simulink model "simulation_Hippocampus_compare_paper"  (R2023a)
settings: Solver=ode3  StartTime=0  StopTime=120  FixedStep=0.001  MaxStep=0.001  MinStep=0.00001  RelTol=1e-5  AbsTol=1e-5  EnableMultiTasking=on
values from neighbouring files (symbols this model uses):
  k_pos_ndi = 8    [parameters.m]
  k_vel_ndi = 8    [parameters.m]
  Kf = 6    [parameters.m]
  Kp = 0.01    [parameters.m]
  Kp_p = 30    [parameters.m]
  Kp_pitch = 8    [parameters.m]
  Kp_q = 10    [parameters.m]
  Kp_r = 10    [parameters.m]
  Kp_roll = 10    [parameters.m]
  Kp_u = 8    [parameters.m]
  Kp_yaw = 8    [parameters.m]
  Kq = 5    [parameters.m]
  Kr = 8    [parameters.m]
  Ktau1 = 0.1    [parameters.m]
  Ktau2 = 5    [parameters.m]
  Ktau3 = 5    [parameters.m]
  Ku = 8    [parameters.m]
  p11 = 0.4    [parameters.m]
  p12 = 0.2    [parameters.m]
  p21 = 0.2    [parameters.m]
  p22 = 0.05    [parameters.m]
  p31 = 0.3    [parameters.m]
  p32 = 0.05    [parameters.m]
  p41 = 0.5    [parameters.m]
  p42 = 0.1    [parameters.m]
  p51 = 0.5    [parameters.m]
  p52 = 0.1    [parameters.m]
  p61 = 0.5    [parameters.m]
  p62 = 0.1    [parameters.m]
  Q1 = -8    [simulation_para.m]
  Q2 = -10    [simulation_para.m]
  Q3 = -[0.01,5,8]    [simulation_para.m]
  Q4 = -[0.001,0.1,0.1]    [simulation_para.m]
  r1 = 4    [parameters.m]
  r2 = 6    [parameters.m]
libraries: simulink x8
(part 2 of 7)

== system simulation_Hippocampus_compare_paper/PDPD1/HippCampus1 ==
  input : Inport
  disturbance : Inport  Port=2
  Controls: Angular Velocities : Scope
  Controls: Rotors1 : Scope
  Controls: Torques : Scope
  Display : Display
  Display1 : Display
  HippoCampus : MATLAB Function  TreatAsAtomicUnit=on
  Integrator : Integrator  InitialCondition=[0; 0; 0; 0;0;0;zeros(6,1)]
  Subsystem : Subsystem
  Subsystem1 : Subsystem
  Subsystem4 : Subsystem
  Sum : Sum  Inputs=|++
  To Workspace8 : ToWorkspace  VariableName=u_PDPD  SaveFormat=Timeseries  SampleTime=-1
  state : Outport
  wires:
  HippoCampus/1(dx) -> Sum/1  "dx"
  Sum/1 -> Integrator/1
  ? -> Controls: Angular Velocities/1
  disturbance/1 -> Sum/2
  Integrator/1 -> Subsystem/1(In1)
  Subsystem/1(state) -> state/1, HippoCampus/1(x)
  Subsystem4/1(Out1) -> Display1/1
  Subsystem1/1(Out1) -> Display/1
  input/1 -> Subsystem4/1(u), To Workspace8/1, Subsystem1/1(u), HippoCampus/2(in), Controls: Torques/1, Controls: Rotors1/1

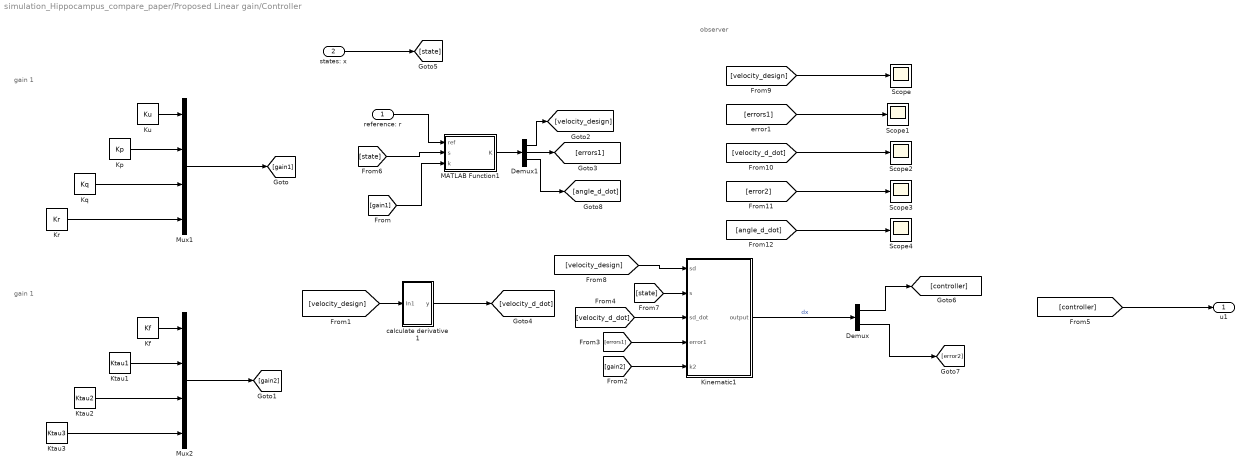
== system simulation_Hippocampus_compare_paper/Proposed Linear gain/Controller ==
  note: observer
  note: gain 1
  note: gain 1
  reference: r : Inport
  states: x : Inport  Port=2
  Demux : Demux  Outputs=[4 4]
  Demux1 : Demux  Outputs=[4 4 2]
  Kf : Constant  Value=Kf
  Kinematic1 : MATLAB Function  TreatAsAtomicUnit=on
  Kp : Constant  Value=Kp
  Kq : Constant  Value=Kq
  Kr : Constant  Value=Kr
  Ktau1 : Constant  Value=Ktau1
  Ktau2 : Constant  Value=Ktau2
  Ktau3 : Constant  Value=Ktau3
  Ku : Constant  Value=Ku
  MATLAB Function1 : MATLAB Function  TreatAsAtomicUnit=on
  Mux1 : Mux
  Mux2 : Mux
  Scope{,1..4} (5 alike) : Scope
  calculate derivative 1 : Subsystem
  u1 : Outport
  wires:
  Kinematic1/1(output) -> Demux/1  "dx"
  [state] -> Kinematic1/2(s)
  reference: r/1 -> MATLAB Function1/1(ref)
  states: x/1 -> [state]
  Ku/1 -> Mux1/1
  Kp/1 -> Mux1/2
  Kq/1 -> Mux1/3
  Kr/1 -> Mux1/4
  Mux1/1 -> [gain1]
  [gain1] -> MATLAB Function1/3(k)
  Ktau3/1 -> Mux2/4
  Ktau1/1 -> Mux2/2
  Ktau2/1 -> Mux2/3
  Mux2/1 -> [gain2]
  Kf/1 -> Mux2/1
  Demux1/1 -> [velocity_design]
  MATLAB Function1/1(K) -> Demux1/1
  Demux1/2 -> [errors1]
  [velocity_design] -> calculate derivative 1/1(In1)
  [gain2] -> Kinematic1/5(k2)
  [errors1] -> Kinematic1/4(error1)
  [state] -> MATLAB Function1/2(s)
  [velocity_design] -> Kinematic1/1(sd)
  Demux/1 -> [controller]
  Demux/2 -> [error2]
  [controller] -> u1/1
  [velocity_design] -> Scope/1
  [errors1] -> Scope1/1
  [velocity_d_dot] -> Scope2/1
  [error2] -> Scope3/1
  calculate derivative 1/1(y) -> [velocity_d_dot]
  Demux1/3 -> [angle_d_dot]
  [angle_d_dot] -> Scope4/1
  [velocity_d_dot] -> Kinematic1/3(sd_dot)

== system simulation_Hippocampus_compare_paper/Proposed Linear gain/Disturbance: All derivatives1 ==
  a : Inport
  a1 : Inport  Port=2
  Input : Inport  Port=3
  Gain1 : Gain  Gain=0  Multiplication=Matrix(K*u)
  Gain2 : Gain  Multiplication=Matrix(K*u)
  Gain3 : Gain  Gain=0  Multiplication=Matrix(K*u)
  MATLAB Function : MATLAB Function  TreatAsAtomicUnit=on
  Sum2 : Sum  Inputs=|+++
  disturbance2 : Subsystem
  disturbance3 : Subsystem
  old disturbance : Subsystem
  disturbance : Outport
  wires:
  Sum2/1 -> MATLAB Function/1(u)
  Gain1/1 -> Sum2/1
  disturbance2/1(Out1) -> Gain2/1
  a/1 -> disturbance3/1(a)
  a1/1 -> disturbance3/2(a1)
  disturbance3/1(d) -> Gain1/1
  Gain2/1 -> Sum2/2
  old disturbance/1(Out1) -> Gain3/1
  Gain3/1 -> Sum2/3
  MATLAB Function/1(y) -> disturbance/1
  Input/1 -> MATLAB Function/2(d)

== system simulation_Hippocampus_compare_paper/Proposed Linear gain/Disturbance: All derivatives2 ==
  a : Inport
  a1 : Inport  Port=2
  Input : Inport  Port=3
  Input1 : Inport  Port=4
  Gain1 : Gain  Gain=0  Multiplication=Matrix(K*u)
  Gain2 : Gain  Multiplication=Matrix(K*u)
  Gain3 : Gain  Gain=0  Multiplication=Matrix(K*u)
  Gain4 : Gain  Gain=0  Multiplication=Matrix(K*u)
  MATLAB Function : MATLAB Function  TreatAsAtomicUnit=on
  MATLAB Function1 : MATLAB Function  TreatAsAtomicUnit=on
  Scope : Scope
  Sum2 : Sum  Inputs=|++++
  disturbance2 : Subsystem
  disturbance3 : Subsystem
  old disturbance : Subsystem
  disturbance : Outport
  wires:
  Sum2/1 -> MATLAB Function/1(u)
  Gain1/1 -> Sum2/1
  disturbance2/1(Out1) -> Gain2/1
  a/1 -> disturbance3/1(a)
  a1/1 -> disturbance3/2(a1)
  disturbance3/1(d) -> Gain1/1
  Gain2/1 -> Sum2/2
  old disturbance/1(Out1) -> Gain3/1
  Gain3/1 -> Sum2/3
  MATLAB Function/1(y) -> disturbance/1
  Input/1 -> MATLAB Function/2(d)
  Input1/1 -> MATLAB Function1/1(u)
  MATLAB Function1/1(d) -> Scope/1, Gain4/1
  Gain4/1 -> Sum2/4

== system simulation_Hippocampus_compare_paper/Proposed Linear gain/HippCampus ==
  input : Inport
  disturbance : Inport  Port=2
  Controls: Rotors1 : Scope
  Controls: Torques : Scope
  Display : Display
  Display1 : Display
  HippoCampus : MATLAB Function  TreatAsAtomicUnit=on
  Integrator : Integrator  InitialCondition=[0; 0; 0; 0;0;0;zeros(6,1)]
  Scope : Scope
  Subsystem : Subsystem
  Subsystem1 : Subsystem
  Subsystem4 : Subsystem
  Sum : Sum  Inputs=|++
  To Workspace7 : ToWorkspace  VariableName=LYAL_u  SaveFormat=Timeseries  SampleTime=-1
  sat1 : MATLAB Function  TreatAsAtomicUnit=on
  state : Outport
  wires:
  HippoCampus/1(dx) -> Sum/1  "dx"
  Sum/1 -> Integrator/1
  disturbance/1 -> Sum/2
  Integrator/1 -> Subsystem/1(In1)
  Subsystem/1(state) -> state/1, HippoCampus/1(x)
  Subsystem4/1(Out1) -> Display1/1
  Subsystem1/1(Out1) -> Display/1
  sat1/1(u_sat) -> Controls: Rotors1/1, Controls: Torques/1, Scope/1, HippoCampus/2(in), Subsystem1/1(u), Subsystem4/1(u), To Workspace7/1
  input/1 -> sat1/1(u)

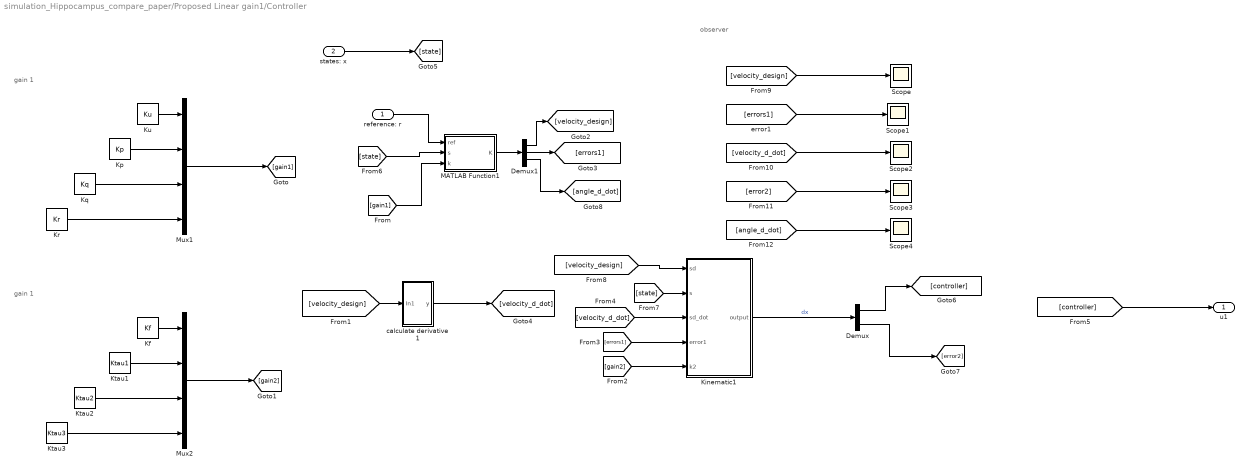
== system simulation_Hippocampus_compare_paper/Proposed Linear gain1/Controller ==
  note: observer
  note: gain 1
  note: gain 1
  reference: r : Inport
  states: x : Inport  Port=2
  Demux : Demux  Outputs=[4 4]
  Demux1 : Demux  Outputs=[4 4 2]
  Kf : Constant  Value=Kf
  Kinematic1 : MATLAB Function  TreatAsAtomicUnit=on
  Kp : Constant  Value=Kp
  Kq : Constant  Value=Kq
  Kr : Constant  Value=Kr
  Ktau1 : Constant  Value=Ktau1
  Ktau2 : Constant  Value=Ktau2
  Ktau3 : Constant  Value=Ktau3
  Ku : Constant  Value=Ku
  MATLAB Function1 : MATLAB Function  TreatAsAtomicUnit=on
  Mux1 : Mux
  Mux2 : Mux
  Scope{,1..4} (5 alike) : Scope
  calculate derivative 1 : Subsystem
  u1 : Outport
  wires:
  Kinematic1/1(output) -> Demux/1  "dx"
  [state] -> Kinematic1/2(s)
  reference: r/1 -> MATLAB Function1/1(ref)
  states: x/1 -> [state]
  Ku/1 -> Mux1/1
  Kp/1 -> Mux1/2
  Kq/1 -> Mux1/3
  Kr/1 -> Mux1/4
  Mux1/1 -> [gain1]
  [gain1] -> MATLAB Function1/3(k)
  Ktau3/1 -> Mux2/4
  Ktau1/1 -> Mux2/2
  Ktau2/1 -> Mux2/3
  Mux2/1 -> [gain2]
  Kf/1 -> Mux2/1
  Demux1/1 -> [velocity_design]
  MATLAB Function1/1(K) -> Demux1/1
  Demux1/2 -> [errors1]
  [velocity_design] -> calculate derivative 1/1(In1)
  [gain2] -> Kinematic1/5(k2)
  [errors1] -> Kinematic1/4(error1)
  [state] -> MATLAB Function1/2(s)
  [velocity_design] -> Kinematic1/1(sd)
  Demux/1 -> [controller]
  Demux/2 -> [error2]
  [controller] -> u1/1
  [velocity_design] -> Scope/1
  [errors1] -> Scope1/1
  [velocity_d_dot] -> Scope2/1
  [error2] -> Scope3/1
  calculate derivative 1/1(y) -> [velocity_d_dot]
  Demux1/3 -> [angle_d_dot]
  [angle_d_dot] -> Scope4/1
  [velocity_d_dot] -> Kinematic1/3(sd_dot)

== system simulation_Hippocampus_compare_paper/Proposed Linear gain1/Disturbance: All derivatives1 ==
  a : Inport
  a1 : Inport  Port=2
  Input : Inport  Port=3
  Gain1 : Gain  Gain=0  Multiplication=Matrix(K*u)
  Gain2 : Gain  Multiplication=Matrix(K*u)
  Gain3 : Gain  Gain=0  Multiplication=Matrix(K*u)
  MATLAB Function : MATLAB Function  TreatAsAtomicUnit=on
  Sum2 : Sum  Inputs=|+++
  disturbance2 : Subsystem
  disturbance3 : Subsystem
  old disturbance : Subsystem
  disturbance : Outport
  wires:
  Sum2/1 -> MATLAB Function/1(u)
  Gain1/1 -> Sum2/1
  disturbance2/1(Out1) -> Gain2/1
  a/1 -> disturbance3/1(a)
  a1/1 -> disturbance3/2(a1)
  disturbance3/1(d) -> Gain1/1
  Gain2/1 -> Sum2/2
  old disturbance/1(Out1) -> Gain3/1
  Gain3/1 -> Sum2/3
  MATLAB Function/1(y) -> disturbance/1
  Input/1 -> MATLAB Function/2(d)

== system simulation_Hippocampus_compare_paper/Proposed Linear gain1/HippCampus ==
  input : Inport
  disturbance : Inport  Port=2
  Controls: Rotors1 : Scope
  Controls: Torques : Scope
  Display : Display
  Display1 : Display
  HippoCampus : MATLAB Function  TreatAsAtomicUnit=on
  Integrator : Integrator  InitialCondition=[0; 0; 0; 0;0;0;zeros(6,1)]
  Scope : Scope
  Subsystem : Subsystem
  Subsystem1 : Subsystem
  Subsystem4 : Subsystem
  Sum : Sum  Inputs=|++
  To Workspace7 : ToWorkspace  VariableName=LYAL_u  SaveFormat=Timeseries  SampleTime=-1
  state : Outport
  wires:
  HippoCampus/1(dx) -> Sum/1  "dx"
  Sum/1 -> Integrator/1
  disturbance/1 -> Sum/2
  Integrator/1 -> Subsystem/1(In1)
  Subsystem/1(state) -> state/1, HippoCampus/1(x)
  Subsystem4/1(Out1) -> Display1/1
  Subsystem1/1(Out1) -> Display/1
  input/1 -> Controls: Rotors1/1, Controls: Torques/1, Scope/1, HippoCampus/2(in), Subsystem1/1(u), Subsystem4/1(u), To Workspace7/1

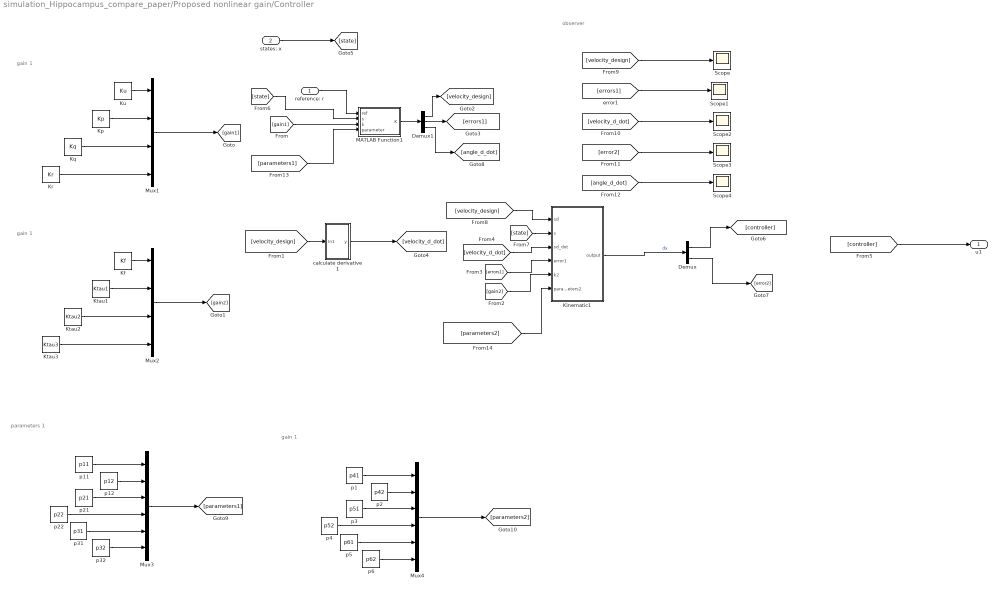
== system simulation_Hippocampus_compare_paper/Proposed nonlinear gain/Controller ==
  note: observer
  note: gain 1
  note: gain 1
  note: parameters 1
  note: gain 1
  reference: r : Inport
  states: x : Inport  Port=2
  Demux : Demux  Outputs=[4 4]
  Demux1 : Demux  Outputs=[4 4 2]
  Kf : Constant  Value=Kf
  Kinematic1 : MATLAB Function  TreatAsAtomicUnit=on
  Kp : Constant  Value=Kp
  Kq : Constant  Value=Kq
  Kr : Constant  Value=Kr
  Ktau1 : Constant  Value=Ktau1
  Ktau2 : Constant  Value=Ktau2
  Ktau3 : Constant  Value=Ktau3
  Ku : Constant  Value=Ku
  MATLAB Function1 : MATLAB Function  TreatAsAtomicUnit=on
  Mux1 : Mux
  Mux2 : Mux
  Mux3 : Mux  Inputs=6
  Mux4 : Mux  Inputs=6
  Scope{,1..4} (5 alike) : Scope
  calculate derivative 1 : Subsystem
  p1 : Constant  Value=p41
  p11 : Constant  Value=p11
  p12 : Constant  Value=p12
  p2 : Constant  Value=p42
  p21 : Constant  Value=p21
  p22 : Constant  Value=p22
  p3 : Constant  Value=p51
  p31 : Constant  Value=p31
  p32 : Constant  Value=p32
  p4 : Constant  Value=p52
  p5 : Constant  Value=p61
  p6 : Constant  Value=p62
  u1 : Outport
  wires:
  Kinematic1/1(output) -> Demux/1  "dx"
  [state] -> Kinematic1/2(s)
  reference: r/1 -> MATLAB Function1/1(ref)
  states: x/1 -> [state]
  Ku/1 -> Mux1/1
  Kp/1 -> Mux1/2
  Kq/1 -> Mux1/3
  Kr/1 -> Mux1/4
  Mux1/1 -> [gain1]
  [gain1] -> MATLAB Function1/3(k)
  Ktau3/1 -> Mux2/4
  Ktau1/1 -> Mux2/2
  Ktau2/1 -> Mux2/3
  Mux2/1 -> [gain2]
  Kf/1 -> Mux2/1
  Demux1/1 -> [velocity_design]
  MATLAB Function1/1(K) -> Demux1/1
  Demux1/2 -> [errors1]
  [velocity_design] -> calculate derivative 1/1(In1)
  [gain2] -> Kinematic1/5(k2)
  [errors1] -> Kinematic1/4(error1)
  [state] -> MATLAB Function1/2(s)
  [velocity_design] -> Kinematic1/1(sd)
  Demux/1 -> [controller]
  Demux/2 -> [error2]
  [controller] -> u1/1
  [velocity_design] -> Scope/1
  [errors1] -> Scope1/1
  [velocity_d_dot] -> Scope2/1
  [error2] -> Scope3/1
  calculate derivative 1/1(y) -> [velocity_d_dot]
  Demux1/3 -> [angle_d_dot]
  [angle_d_dot] -> Scope4/1
  [velocity_d_dot] -> Kinematic1/3(sd_dot)
  p22/1 -> Mux3/4
  p12/1 -> Mux3/2
  p21/1 -> Mux3/3
  Mux3/1 -> [parameters1]
  p11/1 -> Mux3/1
  p31/1 -> Mux3/5
  p32/1 -> Mux3/6
  [parameters1] -> MATLAB Function1/4(parameter)
  Mux4/1 -> [parameters2]
  p5/1 -> Mux4/5
  p6/1 -> Mux4/6
  p3/1 -> Mux4/3
  p2/1 -> Mux4/2
  p4/1 -> Mux4/4
  p1/1 -> Mux4/1
  [parameters2] -> Kinematic1/6(parameters2)

== system simulation_Hippocampus_compare_paper/Proposed nonlinear gain/Disturbance: All derivatives1 ==
  a : Inport
  a1 : Inport  Port=2
  Input : Inport  Port=3
  Input1 : Inport  Port=4
  Gain1 : Gain  Gain=0  Multiplication=Matrix(K*u)
  Gain2 : Gain  Multiplication=Matrix(K*u)
  Gain3 : Gain  Gain=0  Multiplication=Matrix(K*u)
  Gain4 : Gain  Gain=0  Multiplication=Matrix(K*u)
  MATLAB Function : MATLAB Function  TreatAsAtomicUnit=on
  MATLAB Function1 : MATLAB Function  TreatAsAtomicUnit=on
  Scope : Scope
  Sum2 : Sum  Inputs=|++++
  disturbance2 : Subsystem
  disturbance3 : Subsystem
  old disturbance : Subsystem
  disturbance : Outport
  wires:
  Sum2/1 -> MATLAB Function/1(u)
  Gain1/1 -> Sum2/1
  disturbance2/1(Out1) -> Gain2/1
  a/1 -> disturbance3/1(a)
  a1/1 -> disturbance3/2(a1)
  disturbance3/1(d) -> Gain1/1
  Gain2/1 -> Sum2/2
  old disturbance/1(Out1) -> Gain3/1
  Gain3/1 -> Sum2/3
  MATLAB Function/1(y) -> disturbance/1
  Input/1 -> MATLAB Function/2(d)
  Input1/1 -> MATLAB Function1/1(u)
  MATLAB Function1/1(d) -> Scope/1, Gain4/1
  Gain4/1 -> Sum2/4

== system simulation_Hippocampus_compare_paper/Proposed nonlinear gain/HippCampus ==
  input : Inport
  disturbance : Inport  Port=2
  Controls: Angular Velocities : Scope
  Controls: Rotors1 : Scope
  Controls: Torques : Scope
  Display : Display
  Display1 : Display
  HippoCampus : MATLAB Function  TreatAsAtomicUnit=on
  Integrator : Integrator  InitialCondition=[0; 0; 0; 0;0;0;zeros(6,1)]
  Scope : Scope
  Scope1 : Scope
  Subsystem : Subsystem
  Subsystem1 : Subsystem
  Subsystem4 : Subsystem
  Sum : Sum  Inputs=|++
  To Workspace7 : ToWorkspace  VariableName=u  SaveFormat=Timeseries  SampleTime=-1
  sat1 : MATLAB Function  TreatAsAtomicUnit=on
  state : Outport
  wires:
  HippoCampus/1(dx) -> Sum/1  "dx"
  Sum/1 -> Integrator/1
  ? -> Controls: Angular Velocities/1
  disturbance/1 -> Sum/2
  Integrator/1 -> Subsystem/1(In1)
  Subsystem/1(state) -> state/1, HippoCampus/1(x)
  Subsystem4/1(Out1) -> Display1/1
  Subsystem1/1(Out1) -> Display/1
  input/1 -> sat1/1(u)
  sat1/2(omega) -> Scope1/1
  sat1/1(u_sat) -> Controls: Rotors1/1, Controls: Torques/1, Scope/1, HippoCampus/2(in), Subsystem1/1(u), Subsystem4/1(u), To Workspace7/1

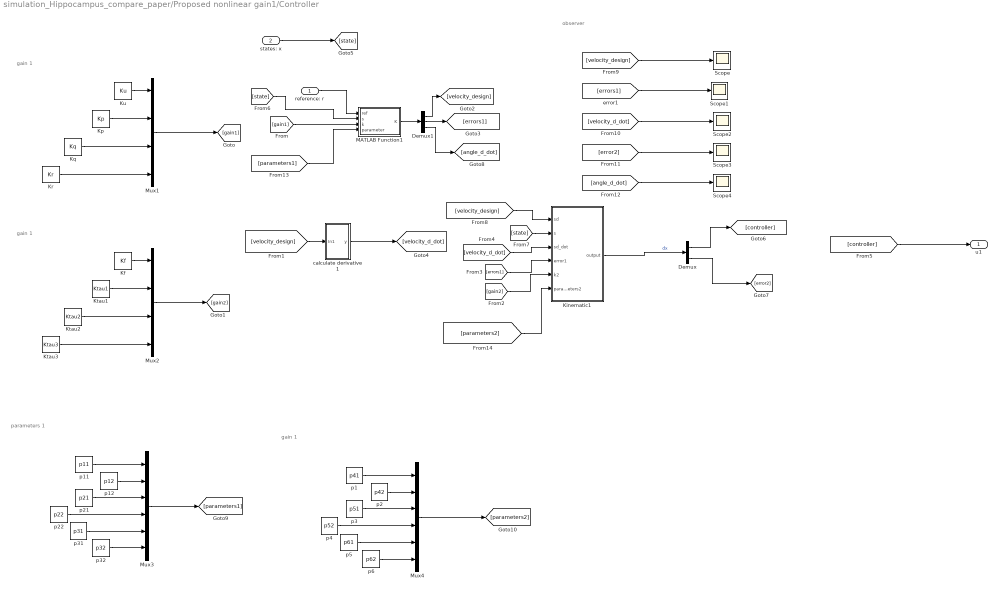
== system simulation_Hippocampus_compare_paper/Proposed nonlinear gain1/Controller ==
  note: observer
  note: gain 1
  note: gain 1
  note: parameters 1
  note: gain 1
  reference: r : Inport
  states: x : Inport  Port=2
  Demux : Demux  Outputs=[4 4]
  Demux1 : Demux  Outputs=[4 4 2]
  Kf : Constant  Value=Kf
  Kinematic1 : MATLAB Function  TreatAsAtomicUnit=on
  Kp : Constant  Value=Kp
  Kq : Constant  Value=Kq
  Kr : Constant  Value=Kr
  Ktau1 : Constant  Value=Ktau1
  Ktau2 : Constant  Value=Ktau2
  Ktau3 : Constant  Value=Ktau3
  Ku : Constant  Value=Ku
  MATLAB Function1 : MATLAB Function  TreatAsAtomicUnit=on
  Mux1 : Mux
  Mux2 : Mux
  Mux3 : Mux  Inputs=6
  Mux4 : Mux  Inputs=6
  Scope{,1..4} (5 alike) : Scope
  calculate derivative 1 : Subsystem
  p1 : Constant  Value=p41
  p11 : Constant  Value=p11
  p12 : Constant  Value=p12
  p2 : Constant  Value=p42
  p21 : Constant  Value=p21
  p22 : Constant  Value=p22
  p3 : Constant  Value=p51
  p31 : Constant  Value=p31
  p32 : Constant  Value=p32
  p4 : Constant  Value=p52
  p5 : Constant  Value=p61
  p6 : Constant  Value=p62
  u1 : Outport
  wires:
  Kinematic1/1(output) -> Demux/1  "dx"
  [state] -> Kinematic1/2(s)
  reference: r/1 -> MATLAB Function1/1(ref)
  states: x/1 -> [state]
  Ku/1 -> Mux1/1
  Kp/1 -> Mux1/2
  Kq/1 -> Mux1/3
  Kr/1 -> Mux1/4
  Mux1/1 -> [gain1]
  [gain1] -> MATLAB Function1/3(k)
  Ktau3/1 -> Mux2/4
  Ktau1/1 -> Mux2/2
  Ktau2/1 -> Mux2/3
  Mux2/1 -> [gain2]
  Kf/1 -> Mux2/1
  Demux1/1 -> [velocity_design]
  MATLAB Function1/1(K) -> Demux1/1
  Demux1/2 -> [errors1]
  [velocity_design] -> calculate derivative 1/1(In1)
  [gain2] -> Kinematic1/5(k2)
  [errors1] -> Kinematic1/4(error1)
  [state] -> MATLAB Function1/2(s)
  [velocity_design] -> Kinematic1/1(sd)
  Demux/1 -> [controller]
  Demux/2 -> [error2]
  [controller] -> u1/1
  [velocity_design] -> Scope/1
  [errors1] -> Scope1/1
  [velocity_d_dot] -> Scope2/1
  [error2] -> Scope3/1
  calculate derivative 1/1(y) -> [velocity_d_dot]
  Demux1/3 -> [angle_d_dot]
  [angle_d_dot] -> Scope4/1
  [velocity_d_dot] -> Kinematic1/3(sd_dot)
  p22/1 -> Mux3/4
  p12/1 -> Mux3/2
  p21/1 -> Mux3/3
  Mux3/1 -> [parameters1]
  p11/1 -> Mux3/1
  p31/1 -> Mux3/5
  p32/1 -> Mux3/6
  [parameters1] -> MATLAB Function1/4(parameter)
  Mux4/1 -> [parameters2]
  p5/1 -> Mux4/5
  p6/1 -> Mux4/6
  p3/1 -> Mux4/3
  p2/1 -> Mux4/2
  p4/1 -> Mux4/4
  p1/1 -> Mux4/1
  [parameters2] -> Kinematic1/6(parameters2)

== system simulation_Hippocampus_compare_paper/Proposed nonlinear gain1/Disturbance: All derivatives1 ==
  a : Inport
  a1 : Inport  Port=2
  Input : Inport  Port=3
  Gain1 : Gain  Gain=0  Multiplication=Matrix(K*u)
  Gain2 : Gain  Multiplication=Matrix(K*u)
  Gain3 : Gain  Gain=0  Multiplication=Matrix(K*u)
  MATLAB Function : MATLAB Function  TreatAsAtomicUnit=on
  Sum2 : Sum  Inputs=|+++
  disturbance2 : Subsystem
  disturbance3 : Subsystem
  old disturbance : Subsystem
  disturbance : Outport
  wires:
  Sum2/1 -> MATLAB Function/1(u)
  Gain1/1 -> Sum2/1
  disturbance2/1(Out1) -> Gain2/1
  a/1 -> disturbance3/1(a)
  a1/1 -> disturbance3/2(a1)
  disturbance3/1(d) -> Gain1/1
  Gain2/1 -> Sum2/2
  old disturbance/1(Out1) -> Gain3/1
  Gain3/1 -> Sum2/3
  MATLAB Function/1(y) -> disturbance/1
  Input/1 -> MATLAB Function/2(d)

== system simulation_Hippocampus_compare_paper/Proposed nonlinear gain1/HippCampus ==
  input : Inport
  disturbance : Inport  Port=2
  Controls: Angular Velocities : Scope
  Controls: Rotors1 : Scope
  Controls: Torques : Scope
  Display : Display
  Display1 : Display
  HippoCampus : MATLAB Function  TreatAsAtomicUnit=on
  Integrator : Integrator  InitialCondition=[0; 0; 0; 0;0;0;zeros(6,1)]
  Scope : Scope
  Subsystem : Subsystem
  Subsystem1 : Subsystem
  Subsystem4 : Subsystem
  Sum : Sum  Inputs=|++
  To Workspace7 : ToWorkspace  VariableName=u  SaveFormat=Timeseries  SampleTime=-1
  state : Outport
  wires:
  HippoCampus/1(dx) -> Sum/1  "dx"
  Sum/1 -> Integrator/1
  ? -> Controls: Angular Velocities/1
  disturbance/1 -> Sum/2
  Integrator/1 -> Subsystem/1(In1)
  Subsystem/1(state) -> state/1, HippoCampus/1(x)
  Subsystem4/1(Out1) -> Display1/1
  Subsystem1/1(Out1) -> Display/1
  input/1 -> Controls: Rotors1/1, Controls: Torques/1, Scope/1, HippoCampus/2(in), Subsystem1/1(u), Subsystem4/1(u), To Workspace7/1

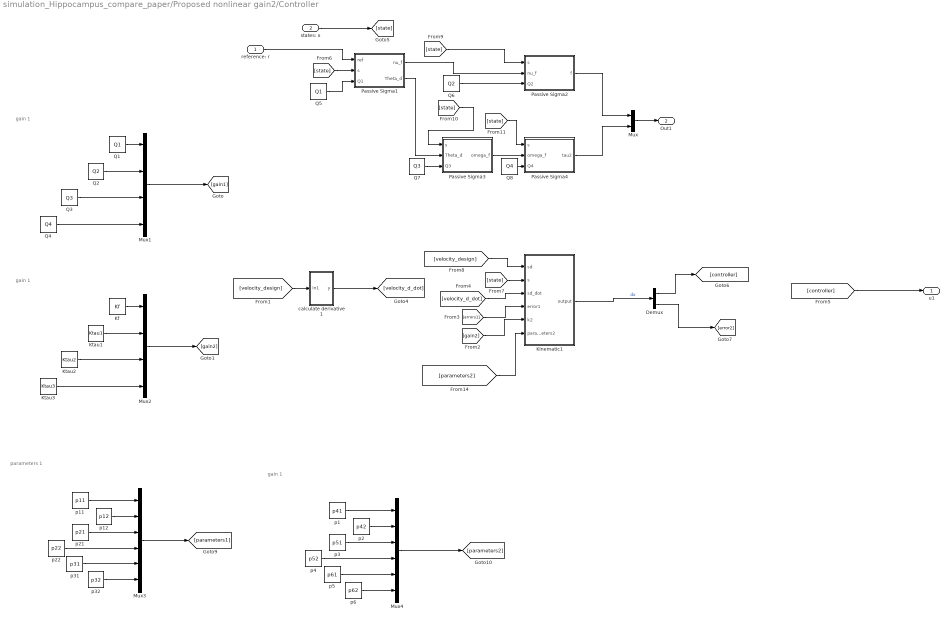
== system simulation_Hippocampus_compare_paper/Proposed nonlinear gain2/Controller ==
  note: gain 1
  note: gain 1
  note: parameters 1
  note: gain 1
  reference: r : Inport
  states: x : Inport  Port=2
  Demux : Demux  Outputs=[4 4]
  Kf : Constant  Value=Kf
  Kinematic1 : MATLAB Function  TreatAsAtomicUnit=on
  Ktau1 : Constant  Value=Ktau1
  Ktau2 : Constant  Value=Ktau2
  Ktau3 : Constant  Value=Ktau3
  Mux : Mux  Inputs=2
  Mux1 : Mux
  Mux2 : Mux
  Mux3 : Mux  Inputs=6
  Mux4 : Mux  Inputs=6
  Passive Sigma1 : MATLAB Function  TreatAsAtomicUnit=on
  Passive Sigma2 : MATLAB Function  TreatAsAtomicUnit=on
  Passive Sigma3 : MATLAB Function  TreatAsAtomicUnit=on
  Passive Sigma4 : MATLAB Function  TreatAsAtomicUnit=on
  Q1 : Constant  Value=Q1
  Q2 : Constant  Value=Q2
  Q3 : Constant  Value=Q3
  Q4 : Constant  Value=Q4
  Q5 : Constant  Value=Q1
  Q6 : Constant  Value=Q2
  Q7 : Constant  Value=Q3
  Q8 : Constant  Value=Q4
  calculate derivative 1 : Subsystem
  p1 : Constant  Value=p41
  p11 : Constant  Value=p11
  p12 : Constant  Value=p12
  p2 : Constant  Value=p42
  p21 : Constant  Value=p21
  p22 : Constant  Value=p22
  p3 : Constant  Value=p51
  p31 : Constant  Value=p31
  p32 : Constant  Value=p32
  p4 : Constant  Value=p52
  p5 : Constant  Value=p61
  p6 : Constant  Value=p62
  u1 : Outport
  Out1 : Outport  Port=2
  wires:
  Kinematic1/1(output) -> Demux/1  "dx"
  [state] -> Kinematic1/2(s)
  reference: r/1 -> Passive Sigma1/1(ref)
  states: x/1 -> [state]
  Q1/1 -> Mux1/1
  Q2/1 -> Mux1/2
  Q3/1 -> Mux1/3
  Q4/1 -> Mux1/4
  Mux1/1 -> [gain1]
  Q5/1 -> Passive Sigma1/3(Q1)
  Ktau3/1 -> Mux2/4
  Ktau1/1 -> Mux2/2
  Ktau2/1 -> Mux2/3
  Mux2/1 -> [gain2]
  Kf/1 -> Mux2/1
  [velocity_design] -> calculate derivative 1/1(In1)
  [gain2] -> Kinematic1/5(k2)
  [errors1] -> Kinematic1/4(error1)
  [state] -> Passive Sigma1/2(s)
  [velocity_design] -> Kinematic1/1(sd)
  Demux/1 -> [controller]
  Demux/2 -> [error2]
  [controller] -> u1/1
  calculate derivative 1/1(y) -> [velocity_d_dot]
  [velocity_d_dot] -> Kinematic1/3(sd_dot)
  p22/1 -> Mux3/4
  p12/1 -> Mux3/2
  p21/1 -> Mux3/3
  Mux3/1 -> [parameters1]
  p11/1 -> Mux3/1
  p31/1 -> Mux3/5
  p32/1 -> Mux3/6
  Mux4/1 -> [parameters2]
  p5/1 -> Mux4/5
  p6/1 -> Mux4/6
  p3/1 -> Mux4/3
  p2/1 -> Mux4/2
  p4/1 -> Mux4/4
  p1/1 -> Mux4/1
  [parameters2] -> Kinematic1/6(parameters2)
  Passive Sigma1/1(nu_f) -> Passive Sigma2/2(nu_f)
  [state] -> Passive Sigma2/1(s)
  [state] -> Passive Sigma3/1(s)
  Passive Sigma1/2(Theta_d) -> Passive Sigma3/2(Theta_d)
  Passive Sigma3/1(omega_f) -> Passive Sigma4/2(omega_f)
  [state] -> Passive Sigma4/1(s)
  Q6/1 -> Passive Sigma2/3(Q2)
  Q7/1 -> Passive Sigma3/3(Q3)
  Q8/1 -> Passive Sigma4/3(Q4)
  Passive Sigma2/1(f) -> Mux/1
  Passive Sigma4/1(tau2) -> Mux/2
  Mux/1 -> Out1/1

== system simulation_Hippocampus_compare_paper/Proposed nonlinear gain2/HippCampus ==
  input : Inport
  disturbance : Inport  Port=2
  Controls: Angular Velocities : Scope
  Controls: Rotors1 : Scope
  Controls: Torques : Scope
  Display : Display
  Display1 : Display
  HippoCampus : MATLAB Function  TreatAsAtomicUnit=on
  Integrator : Integrator  InitialCondition=[0; 0; 0; 0;0;0;zeros(6,1)]
  Scope : Scope
  Scope1 : Scope
  Subsystem : Subsystem
  Subsystem1 : Subsystem
  Subsystem4 : Subsystem
  Sum : Sum  Inputs=|++
  To Workspace7 : ToWorkspace  VariableName=u  SaveFormat=Timeseries  SampleTime=-1
  sat1 : MATLAB Function  TreatAsAtomicUnit=on
  state : Outport
  wires:
  HippoCampus/1(dx) -> Sum/1  "dx"
  Sum/1 -> Integrator/1
  ? -> Controls: Angular Velocities/1
  disturbance/1 -> Sum/2
  Integrator/1 -> Subsystem/1(In1)
  Subsystem/1(state) -> state/1, HippoCampus/1(x)
  Subsystem4/1(Out1) -> Display1/1
  Subsystem1/1(Out1) -> Display/1
  input/1 -> sat1/1(u)
  sat1/2(omega) -> Scope1/1
  sat1/1(u_sat) -> Controls: Rotors1/1, Controls: Torques/1, Scope/1, HippoCampus/2(in), Subsystem1/1(u), Subsystem4/1(u), To Workspace7/1

== system simulation_Hippocampus_compare_paper/Stabilizing without v w /Controller ==
  note: observer
  note: gain 1
  note: gain 1
  reference: r : Inport
  states: x : Inport  Port=2
  Demux : Demux  Outputs=[4 4]
  Demux1 : Demux  Outputs=[4 4 2]
  Kf : Constant  Value=Kf
  Kinematic1 : MATLAB Function  TreatAsAtomicUnit=on
  Kp : Constant  Value=Kp
  Kq : Constant  Value=Kq
  Kr : Constant  Value=Kr
  Ktau1 : Constant  Value=Ktau1
  Ktau2 : Constant  Value=Ktau2
  Ktau3 : Constant  Value=Ktau3
  Ku : Constant  Value=Ku
  MATLAB Function1 : MATLAB Function  TreatAsAtomicUnit=on
  Mux1 : Mux
  Mux2 : Mux
  Scope{,1..4} (5 alike) : Scope
  calculate derivative 1 : Subsystem
  u1 : Outport
  wires:
  Kinematic1/1(output) -> Demux/1  "dx"
  [state] -> Kinematic1/2(s)
  reference: r/1 -> MATLAB Function1/1(ref)
  states: x/1 -> [state]
  Ku/1 -> Mux1/1
  Kp/1 -> Mux1/2
  Kq/1 -> Mux1/3
  Kr/1 -> Mux1/4
  Mux1/1 -> [gain1]
  [gain1] -> MATLAB Function1/3(k)
  Ktau3/1 -> Mux2/4
  Ktau1/1 -> Mux2/2
  Ktau2/1 -> Mux2/3
  Mux2/1 -> [gain2]
  Kf/1 -> Mux2/1
  Demux1/1 -> [velocity_design]
  MATLAB Function1/1(K) -> Demux1/1
  Demux1/2 -> [errors1]
  [velocity_design] -> calculate derivative 1/1(In1)
  [gain2] -> Kinematic1/5(k2)
  [errors1] -> Kinematic1/4(error1)
  [state] -> MATLAB Function1/2(s)
  [velocity_design] -> Kinematic1/1(sd)
  Demux/1 -> [controller]
  Demux/2 -> [error2]
  [controller] -> u1/1
  [velocity_design] -> Scope/1
  [errors1] -> Scope1/1
  [velocity_d_dot] -> Scope2/1
  [error2] -> Scope3/1
  calculate derivative 1/1(y) -> [velocity_d_dot]
  Demux1/3 -> [angle_d_dot]
  [angle_d_dot] -> Scope4/1
  [velocity_d_dot] -> Kinematic1/3(sd_dot)

== system simulation_Hippocampus_compare_paper/Stabilizing without v w /HippCampus ==
  input : Inport
  disturbance : Inport  Port=2
  Controls: Angular Velocities : Scope
  Controls: Rotors1 : Scope
  Controls: Torques : Scope
  Display : Display
  Display1 : Display
  HippoCampus : MATLAB Function  TreatAsAtomicUnit=on
  Integrator : Integrator  InitialCondition=[0; 0; 0; 0;0;0;zeros(6,1)]
  MATLAB Function : MATLAB Function  TreatAsAtomicUnit=on
  Subsystem : Subsystem
  Subsystem1 : Subsystem
  Subsystem4 : Subsystem
  Sum : Sum  Inputs=|++
  sat1 : MATLAB Function  TreatAsAtomicUnit=on
  state : Outport
  wires:
  HippoCampus/1(dx) -> Sum/1  "dx"
  Sum/1 -> Integrator/1
  ? -> Controls: Angular Velocities/1
  disturbance/1 -> Sum/2
  Integrator/1 -> MATLAB Function/1(u)
  Subsystem4/1(Out1) -> Display1/1
  Subsystem1/1(Out1) -> Display/1
  sat1/1(u_sat) -> Controls: Rotors1/1, Controls: Torques/1, Subsystem1/1(u), HippoCampus/2(in), Subsystem4/1(u)
  MATLAB Function/1(y) -> Subsystem/1(In1)
  Subsystem/1(state) -> state/1, HippoCampus/1(x)
  input/1 -> sat1/1(u)

== system simulation_Hippocampus_compare_paper/Stabilizing without v w 1/Controller ==
  In4 : Inport
  x : Inport  Port=2
  Demux : Demux  Outputs=[4 4]
  Demux4 : Demux  Outputs=[3 3 3 3]
  Kinematic1 : MATLAB Function  TreatAsAtomicUnit=on
  MATLAB Function1 : MATLAB Function  TreatAsAtomicUnit=on
  Mux : Mux  Inputs=2
  Mux1 : Mux  Inputs=2
  Mux2 : Mux  Inputs=3
  Mux3 : Mux  Inputs=3
  Mux8 : Mux  Inputs=2
  Scope : Scope
  Scope1 : Scope
  "calculate derivative " : Subsystem
  u1 : Outport
  wires:
  Demux4/2 -> Mux8/2
  Demux4/1 -> Mux8/1
  x/1 -> Mux3/2, Demux4/1
  Demux4/3 -> Mux1/1
  Demux4/4 -> Mux1/2
  Kinematic1/1(output) -> u1/1  "dx"
  Mux2/1 -> MATLAB Function1/1(s)
  Mux3/1 -> Kinematic1/1(s)
  In4/1 -> Mux2/1
  Mux1/1 -> Mux2/3
  Mux8/1 -> Mux2/2
  MATLAB Function1/1(K) -> Demux/1
  Demux/2 -> Mux/2
  Mux/1 -> Mux3/3, Scope/1
  Demux/1 -> "calculate derivative "/1(In1), Mux3/1, Scope1/1
  "calculate derivative "/1(y) -> Mux/1

== system simulation_Hippocampus_compare_paper/Stabilizing without v w 1/HippCampus ==
  input : Inport
  disturbance : Inport  Port=2
  Controls: Angular Velocities : Scope
  Controls: Rotors1 : Scope
  Controls: Torques : Scope
  Display : Display
  Display1 : Display
  HippoCampus : MATLAB Function  TreatAsAtomicUnit=on
  Integrator : Integrator  InitialCondition=[0; 0; 0; 0;0;0;zeros(6,1)]
  MATLAB Function : MATLAB Function  TreatAsAtomicUnit=on
  Subsystem : Subsystem
  Subsystem1 : Subsystem
  Subsystem4 : Subsystem
  Sum : Sum  Inputs=|++
  sat1 : MATLAB Function  TreatAsAtomicUnit=on
  state : Outport
  wires:
  HippoCampus/1(dx) -> Sum/1  "dx"
  Sum/1 -> Integrator/1
  ? -> Controls: Angular Velocities/1
  disturbance/1 -> Sum/2
  Integrator/1 -> MATLAB Function/1(u)
  Subsystem4/1(Out1) -> Display1/1
  Subsystem1/1(Out1) -> Display/1
  sat1/1(u_sat) -> Controls: Rotors1/1, Controls: Torques/1, Subsystem1/1(u), HippoCampus/2(in), Subsystem4/1(u)
  MATLAB Function/1(y) -> Subsystem/1(In1)
  Subsystem/1(state) -> state/1, HippoCampus/1(x)
  input/1 -> sat1/1(u)

== system simulation_Hippocampus_compare_paper/NDI/Controller/Subsystem ==
  u_ref : Inport
  rpy_ref : Inport  Port=2
  state : Inport  Port=3
  Demux : Demux
  Manual Switch : ManualSwitch
  Mux : Mux  Inputs=2
  Mux1 : Mux
  Scope : Scope
  Subsystem1 : Subsystem
  Subsystem2 : Subsystem
  Terminator : Terminator
  tau : Outport
  wires:
  state/1 -> Subsystem1/2(state), Subsystem2/1(state)
  Subsystem2/1(tau) -> Manual Switch/2, Demux/1
  rpy_ref/1 -> Subsystem1/1(rpy_ref)
  Mux/1 -> Scope/1, Subsystem2/2(upqr_ref)
  u_ref/1 -> Mux1/1, Mux/1
  Demux/2 -> Mux1/2
  Demux/3 -> Mux1/3
  Demux/4 -> Mux1/4
  Manual Switch/1 -> tau/1
  Mux1/1 -> Manual Switch/1
  Demux/1 -> Terminator/1
  Subsystem1/1(pqr_ref) -> Mux/2

== system simulation_Hippocampus_compare_paper/NDI/Controller/Subsystem1 ==
  x : Inport
  Demux1 : Demux  Outputs=12
  MATLAB Function : MATLAB Function  TreatAsAtomicUnit=on
  Mux1 : Mux  Inputs=12
  x_2pi : Outport
  wires:
  Mux1/1 -> x_2pi/1
  x/1 -> Demux1/1
  Demux1/6 -> MATLAB Function/1(u)
  Demux1/1 -> Mux1/1
  Demux1/2 -> Mux1/2
  Demux1/3 -> Mux1/3
  Demux1/4 -> Mux1/4
  Demux1/5 -> Mux1/5
  Demux1/7 -> Mux1/7
  Demux1/8 -> Mux1/8
  Demux1/9 -> Mux1/9
  Demux1/10 -> Mux1/10
  Demux1/11 -> Mux1/11
  Demux1/12 -> Mux1/12
  MATLAB Function/1(y) -> Mux1/6

== system simulation_Hippocampus_compare_paper/NDI/Disturbance: All derivatives1/disturbance2 ==
  Gain : Gain  Gain=[zeros(6,1);ones(6,1)]  Multiplication=Matrix(K*u)
  Step2 : Step  Time=60  After=0.5  SampleTime=0
  Step3 : Step  Time=55  After=0  SampleTime=0
  Sum1 : Sum  Inputs=|++
  Out1 : Outport
  wires:
  Step2/1 -> Sum1/1
  Step3/1 -> Sum1/2
  Gain/1 -> Out1/1
  Sum1/1 -> Gain/1

== system simulation_Hippocampus_compare_paper/NDI/Disturbance: All derivatives1/disturbance3 ==
  a : Inport
  a1 : Inport  Port=2
  Constant : Constant  Value=10
  MATLAB Function : MATLAB Function  TreatAsAtomicUnit=on
  Subsystem : Subsystem
  Subsystem1 : Subsystem
  d : Outport
  wires:
  Subsystem1/1(Out1) -> MATLAB Function/3(u_wave)
  Constant/1 -> MATLAB Function/5(u_un)
  Subsystem/1(Out1) -> MATLAB Function/4(u_c)
  MATLAB Function/1(d) -> d/1
  a1/1 -> MATLAB Function/1(p)
  a/1 -> MATLAB Function/2(a)

== system simulation_Hippocampus_compare_paper/NDI/Disturbance: All derivatives1/old disturbance ==
  Gain : Gain  Gain=ones(12,1)  Multiplication=Matrix(K*u)
  Step : Step  Time=50  After=0.5  SampleTime=0
  Step1 : Step  Time=55  After=-0.5  SampleTime=0
  Step2 : Step  Time=100  After=0.5  SampleTime=0
  Step3 : Step  Time=105  After=-0.5  SampleTime=0
  Sum : Sum  Inputs=|++
  Sum2 : Sum  Inputs=|++
  Sum3 : Sum  Inputs=|++
  Out1 : Outport
  wires:
  Gain/1 -> Out1/1
  Sum3/1 -> Gain/1
  Step3/1 -> Sum2/2
  Step/1 -> Sum/1
  Step1/1 -> Sum/2
  Step2/1 -> Sum2/1
  Sum/1 -> Sum3/1
  Sum2/1 -> Sum3/2

== system simulation_Hippocampus_compare_paper/NDI/Disturbance: All derivatives2/disturbance2 ==
  Gain : Gain  Gain=[0;0;0;0;0;0;1;1;1;1;1;1]  Multiplication=Matrix(K*u)
  Step2 : Step  Time=60  After=0.5  SampleTime=0
  Step3 : Step  Time=55  After=0  SampleTime=0
  Sum1 : Sum
  Out1 : Outport
  wires:
  Step2/1 -> Sum1/1
  Step3/1 -> Sum1/2
  Gain/1 -> Out1/1
  Sum1/1 -> Gain/1

== system simulation_Hippocampus_compare_paper/NDI/Disturbance: All derivatives2/disturbance3 ==
  note: Subsystem
  a : Inport
  a1 : Inport  Port=2
  Constant : Constant  Value=10
  Constant2 : Constant  Value=10
  Constant3 : Constant  Value=45
  Constant4 : Constant  Value=20
  Gain : Gain  Gain=pi/180
  Gain1 : Gain  Gain=pi/180
  MATLAB Function : MATLAB Function  TreatAsAtomicUnit=on
  Mux : Mux  Inputs=3
  Subsystem1 : Subsystem
  d : Outport
  wires:
  Subsystem1/1(Out1) -> MATLAB Function/3(u_wave)
  Constant/1 -> MATLAB Function/5(u_un)
  Mux/1 -> MATLAB Function/4(u_c)
  MATLAB Function/1(d) -> d/1
  a1/1 -> MATLAB Function/1(p)
  a/1 -> MATLAB Function/2(a)
  Constant4/1 -> Mux/1
  Gain/1 -> Mux/2
  Gain1/1 -> Mux/3
  Constant3/1 -> Gain1/1
  Constant2/1 -> Gain/1

== system simulation_Hippocampus_compare_paper/NDI/Disturbance: All derivatives2/old disturbance ==
  Gain : Gain  Gain=ones(12,1)  Multiplication=Matrix(K*u)
  Step : Step  Time=50  After=0.5  SampleTime=0
  Step1 : Step  Time=55  After=-0.5  SampleTime=0
  Step2 : Step  Time=100  After=0.5  SampleTime=0
  Step3 : Step  Time=105  After=-0.5  SampleTime=0
  Sum : Sum  Inputs=|++
  Sum2 : Sum  Inputs=|++
  Sum3 : Sum  Inputs=|++
  Out1 : Outport
  wires:
  Gain/1 -> Out1/1
  Sum3/1 -> Gain/1
  Step3/1 -> Sum2/2
  Step/1 -> Sum/1
  Step1/1 -> Sum/2
  Step2/1 -> Sum2/1
  Sum/1 -> Sum3/1
  Sum2/1 -> Sum3/2

== system simulation_Hippocampus_compare_paper/NDI/HippCampus1/Subsystem ==
  In1 : Inport
  Demux : Demux  Outputs=[5 1 6]
  MATLAB Function : MATLAB Function  TreatAsAtomicUnit=on
  Mux : Mux  Inputs=3
  state : Outport
  wires:
  Demux/2 -> MATLAB Function/1(u)
  MATLAB Function/1(y) -> Mux/2
  In1/1 -> Demux/1
  Demux/3 -> Mux/3
  Demux/1 -> Mux/1
  Mux/1 -> state/1

== system simulation_Hippocampus_compare_paper/NDI/HippCampus1/Subsystem1 ==
  u : Inport
  Integrator2 : Integrator
  Sqrt1 : Sqrt
  norm1 : MATLAB Function  TreatAsAtomicUnit=on
  Out1 : Outport
  wires:
  norm1/1(y) -> Integrator2/1
  Sqrt1/1 -> Out1/1
  Integrator2/1 -> Sqrt1/1
  u/1 -> norm1/1(u)

== system simulation_Hippocampus_compare_paper/NDI/HippCampus1/Subsystem4 ==
  u : Inport
  Demux : Demux
  Mux : Mux
  Subsystem : Subsystem
  Subsystem1 : Subsystem
  Subsystem2 : Subsystem
  Subsystem3 : Subsystem
  Out1 : Outport
  wires:
  Subsystem2/1(Out1) -> Mux/3
  Demux/4 -> Subsystem3/1(u)
  Demux/3 -> Subsystem2/1(u)
  Subsystem1/1(Out1) -> Mux/2
  Demux/2 -> Subsystem1/1(u)
  Subsystem3/1(Out1) -> Mux/4
  Demux/1 -> Subsystem/1(u)
  Subsystem/1(Out1) -> Mux/1
  Mux/1 -> Out1/1
  u/1 -> Demux/1

== system simulation_Hippocampus_compare_paper/NDI4/Controller/Subsystem ==
  u_ref : Inport
  rpy_ref : Inport  Port=2
  state : Inport  Port=3
  Demux : Demux
  Manual Switch : ManualSwitch
  Mux : Mux  Inputs=2
  Mux1 : Mux
  Scope : Scope
  Subsystem1 : Subsystem
  Subsystem2 : Subsystem
  Terminator : Terminator
  tau : Outport
  wires:
  state/1 -> Subsystem1/2(state), Subsystem2/1(state)
  Subsystem1/1(pqr_ref) -> Mux/2
  Subsystem2/1(tau) -> Manual Switch/2, Demux/1
  rpy_ref/1 -> Subsystem1/1(rpy_ref)
  Mux/1 -> Scope/1, Subsystem2/2(upqr_ref)
  u_ref/1 -> Mux1/1, Mux/1
  Demux/2 -> Mux1/2
  Demux/3 -> Mux1/3
  Demux/4 -> Mux1/4
  Manual Switch/1 -> tau/1
  Mux1/1 -> Manual Switch/1
  Demux/1 -> Terminator/1

== system simulation_Hippocampus_compare_paper/NDI4/Controller/Subsystem1 ==
  x : Inport
  Demux1 : Demux  Outputs=12
  MATLAB Function : MATLAB Function  TreatAsAtomicUnit=on
  Mux1 : Mux  Inputs=12
  x_2pi : Outport
  wires:
  Mux1/1 -> x_2pi/1
  x/1 -> Demux1/1
  Demux1/6 -> MATLAB Function/1(u)
  Demux1/1 -> Mux1/1
  Demux1/2 -> Mux1/2
  Demux1/3 -> Mux1/3
  Demux1/4 -> Mux1/4
  Demux1/5 -> Mux1/5
  Demux1/7 -> Mux1/7
  Demux1/8 -> Mux1/8
  Demux1/9 -> Mux1/9
  Demux1/10 -> Mux1/10
  Demux1/11 -> Mux1/11
  Demux1/12 -> Mux1/12
  MATLAB Function/1(y) -> Mux1/6

== system simulation_Hippocampus_compare_paper/NDI4/Disturbance: All derivatives1/disturbance2 ==
  Gain : Gain  Gain=[zeros(6,1);ones(6,1)]  Multiplication=Matrix(K*u)
  Step2 : Step  Time=60  After=0.5  SampleTime=0
  Step3 : Step  Time=55  After=0  SampleTime=0
  Sum1 : Sum  Inputs=|++
  Out1 : Outport
  wires:
  Step2/1 -> Sum1/1
  Step3/1 -> Sum1/2
  Gain/1 -> Out1/1
  Sum1/1 -> Gain/1

== system simulation_Hippocampus_compare_paper/NDI4/Disturbance: All derivatives1/disturbance3 ==
  a : Inport
  a1 : Inport  Port=2
  Constant : Constant  Value=10
  MATLAB Function : MATLAB Function  TreatAsAtomicUnit=on
  Subsystem : Subsystem
  Subsystem1 : Subsystem
  d : Outport
  wires:
  Subsystem1/1(Out1) -> MATLAB Function/3(u_wave)
  Constant/1 -> MATLAB Function/5(u_un)
  Subsystem/1(Out1) -> MATLAB Function/4(u_c)
  MATLAB Function/1(d) -> d/1
  a1/1 -> MATLAB Function/1(p)
  a/1 -> MATLAB Function/2(a)

== system simulation_Hippocampus_compare_paper/NDI4/Disturbance: All derivatives1/old disturbance ==
  Gain : Gain  Gain=ones(12,1)  Multiplication=Matrix(K*u)
  Step : Step  Time=50  After=0.5  SampleTime=0
  Step1 : Step  Time=55  After=-0.5  SampleTime=0
  Step2 : Step  Time=100  After=0.5  SampleTime=0
  Step3 : Step  Time=105  After=-0.5  SampleTime=0
  Sum : Sum  Inputs=|++
  Sum2 : Sum  Inputs=|++
  Sum3 : Sum  Inputs=|++
  Out1 : Outport
  wires:
  Gain/1 -> Out1/1
  Sum3/1 -> Gain/1
  Step3/1 -> Sum2/2
  Step/1 -> Sum/1
  Step1/1 -> Sum/2
  Step2/1 -> Sum2/1
  Sum/1 -> Sum3/1
  Sum2/1 -> Sum3/2

== system simulation_Hippocampus_compare_paper/NDI4/Disturbance: All derivatives2/disturbance2 ==
  Gain : Gain  Gain=[0;0;0;0;0;0;1;1;1;1;1;1]  Multiplication=Matrix(K*u)
  Step2 : Step  Time=60  After=0.5  SampleTime=0
  Step3 : Step  Time=55  After=0  SampleTime=0
  Sum1 : Sum
  Out1 : Outport
  wires:
  Step2/1 -> Sum1/1
  Step3/1 -> Sum1/2
  Gain/1 -> Out1/1
  Sum1/1 -> Gain/1

== system simulation_Hippocampus_compare_paper/NDI4/Disturbance: All derivatives2/disturbance3 ==
  note: Subsystem
  a : Inport
  a1 : Inport  Port=2
  Constant : Constant  Value=10
  Constant2 : Constant  Value=10
  Constant3 : Constant  Value=45
  Constant4 : Constant  Value=20
  Gain : Gain  Gain=pi/180
  Gain1 : Gain  Gain=pi/180
  MATLAB Function : MATLAB Function  TreatAsAtomicUnit=on
  Mux : Mux  Inputs=3
  Subsystem1 : Subsystem
  d : Outport
  wires:
  Subsystem1/1(Out1) -> MATLAB Function/3(u_wave)
  Constant/1 -> MATLAB Function/5(u_un)
  Mux/1 -> MATLAB Function/4(u_c)
  MATLAB Function/1(d) -> d/1
  a1/1 -> MATLAB Function/1(p)
  a/1 -> MATLAB Function/2(a)
  Constant4/1 -> Mux/1
  Gain/1 -> Mux/2
  Gain1/1 -> Mux/3
  Constant3/1 -> Gain1/1
  Constant2/1 -> Gain/1

== system simulation_Hippocampus_compare_paper/NDI4/Disturbance: All derivatives2/old disturbance ==
  Gain : Gain  Gain=ones(12,1)  Multiplication=Matrix(K*u)
  Step : Step  Time=50  After=0.5  SampleTime=0
  Step1 : Step  Time=55  After=-0.5  SampleTime=0
  Step2 : Step  Time=100  After=0.5  SampleTime=0
  Step3 : Step  Time=105  After=-0.5  SampleTime=0
  Sum : Sum  Inputs=|++
  Sum2 : Sum  Inputs=|++
  Sum3 : Sum  Inputs=|++
  Out1 : Outport
  wires:
  Gain/1 -> Out1/1
  Sum3/1 -> Gain/1
  Step3/1 -> Sum2/2
  Step/1 -> Sum/1
  Step1/1 -> Sum/2
  Step2/1 -> Sum2/1
  Sum/1 -> Sum3/1
  Sum2/1 -> Sum3/2

== system simulation_Hippocampus_compare_paper/NDI4/HippCampus1/Subsystem ==
  In1 : Inport
  Demux : Demux  Outputs=[5 1 6]
  MATLAB Function : MATLAB Function  TreatAsAtomicUnit=on
  Mux : Mux  Inputs=3
  state : Outport
  wires:
  Demux/2 -> MATLAB Function/1(u)
  MATLAB Function/1(y) -> Mux/2
  In1/1 -> Demux/1
  Demux/3 -> Mux/3
  Demux/1 -> Mux/1
  Mux/1 -> state/1

== system simulation_Hippocampus_compare_paper/NDI4/HippCampus1/Subsystem1 ==
  u : Inport
  Integrator2 : Integrator
  Sqrt1 : Sqrt
  norm1 : MATLAB Function  TreatAsAtomicUnit=on
  Out1 : Outport
  wires:
  norm1/1(y) -> Integrator2/1
  Sqrt1/1 -> Out1/1
  Integrator2/1 -> Sqrt1/1
  u/1 -> norm1/1(u)

== system simulation_Hippocampus_compare_paper/NDI4/HippCampus1/Subsystem4 ==
  u : Inport
  Demux : Demux
  Mux : Mux
  Subsystem : Subsystem
  Subsystem1 : Subsystem
  Subsystem2 : Subsystem
  Subsystem3 : Subsystem
  Out1 : Outport
  wires:
  Subsystem2/1(Out1) -> Mux/3
  Demux/4 -> Subsystem3/1(u)
  Demux/3 -> Subsystem2/1(u)
  Subsystem1/1(Out1) -> Mux/2
  Demux/2 -> Subsystem1/1(u)
  Subsystem3/1(Out1) -> Mux/4
  Demux/1 -> Subsystem/1(u)
  Subsystem/1(Out1) -> Mux/1
  Mux/1 -> Out1/1
  u/1 -> Demux/1

== system simulation_Hippocampus_compare_paper/PDPD/Controller/Subsystem1 ==
  x : Inport
  Demux1 : Demux  Outputs=12
  MATLAB Function : MATLAB Function  TreatAsAtomicUnit=on
  Mux1 : Mux  Inputs=12
  x_2pi : Outport
  wires:
  Mux1/1 -> x_2pi/1
  x/1 -> Demux1/1
  Demux1/6 -> MATLAB Function/1(u)
  Demux1/1 -> Mux1/1
  Demux1/2 -> Mux1/2
  Demux1/3 -> Mux1/3
  Demux1/4 -> Mux1/4
  Demux1/5 -> Mux1/5
  Demux1/7 -> Mux1/7
  Demux1/8 -> Mux1/8
  Demux1/9 -> Mux1/9
  Demux1/10 -> Mux1/10
  Demux1/11 -> Mux1/11
  Demux1/12 -> Mux1/12
  MATLAB Function/1(y) -> Mux1/6

== system simulation_Hippocampus_compare_paper/PDPD/Disturbance: All derivatives1/disturbance2 ==
  Gain : Gain  Gain=[zeros(6,1);ones(6,1)]  Multiplication=Matrix(K*u)
  Step2 : Step  Time=60  After=0.5  SampleTime=0
  Step3 : Step  Time=55  After=0  SampleTime=0
  Sum1 : Sum
  Out1 : Outport
  wires:
  Step2/1 -> Sum1/1
  Step3/1 -> Sum1/2
  Gain/1 -> Out1/1
  Sum1/1 -> Gain/1

== system simulation_Hippocampus_compare_paper/PDPD/Disturbance: All derivatives1/disturbance3 ==
  note: Subsystem
  a : Inport
  a1 : Inport  Port=2
  Constant : Constant  Value=10
  Constant2 : Constant  Value=10
  Constant3 : Constant  Value=45
  Constant4 : Constant  Value=20
  Gain : Gain  Gain=pi/180
  Gain1 : Gain  Gain=pi/180
  MATLAB Function : MATLAB Function  TreatAsAtomicUnit=on
  Mux : Mux  Inputs=3
  Subsystem1 : Subsystem
  d : Outport
  wires:
  Subsystem1/1(Out1) -> MATLAB Function/3(u_wave)
  Constant/1 -> MATLAB Function/5(u_un)
  Mux/1 -> MATLAB Function/4(u_c)
  MATLAB Function/1(d) -> d/1
  a1/1 -> MATLAB Function/1(p)
  a/1 -> MATLAB Function/2(a)
  Constant4/1 -> Mux/1
  Gain/1 -> Mux/2
  Gain1/1 -> Mux/3
  Constant3/1 -> Gain1/1
  Constant2/1 -> Gain/1

== system simulation_Hippocampus_compare_paper/PDPD/Disturbance: All derivatives1/old disturbance ==
  Gain : Gain  Gain=ones(12,1)  Multiplication=Matrix(K*u)
  Step : Step  Time=50  After=0.5  SampleTime=0
  Step1 : Step  Time=55  After=-0.5  SampleTime=0
  Step2 : Step  Time=100  After=0.5  SampleTime=0
  Step3 : Step  Time=105  After=-0.5  SampleTime=0
  Sum : Sum  Inputs=|++
  Sum2 : Sum  Inputs=|++
  Sum3 : Sum  Inputs=|++
  Out1 : Outport
  wires:
  Gain/1 -> Out1/1
  Sum3/1 -> Gain/1
  Step3/1 -> Sum2/2
  Step/1 -> Sum/1
  Step1/1 -> Sum/2
  Step2/1 -> Sum2/1
  Sum/1 -> Sum3/1
  Sum2/1 -> Sum3/2

== system simulation_Hippocampus_compare_paper/PDPD/HippCampus1/Subsystem ==
  In1 : Inport
  Demux : Demux  Outputs=[5 1 6]
  MATLAB Function : MATLAB Function  TreatAsAtomicUnit=on
  Mux : Mux  Inputs=3
  state : Outport
  wires:
  Demux/2 -> MATLAB Function/1(u)
  MATLAB Function/1(y) -> Mux/2
  In1/1 -> Demux/1
  Demux/3 -> Mux/3
  Demux/1 -> Mux/1
  Mux/1 -> state/1

== system simulation_Hippocampus_compare_paper/PDPD/HippCampus1/Subsystem1 ==
  u : Inport
  Integrator2 : Integrator
  Sqrt1 : Sqrt
  norm1 : MATLAB Function  TreatAsAtomicUnit=on
  Out1 : Outport
  wires:
  norm1/1(y) -> Integrator2/1
  Sqrt1/1 -> Out1/1
  Integrator2/1 -> Sqrt1/1
  u/1 -> norm1/1(u)

== system simulation_Hippocampus_compare_paper/PDPD/HippCampus1/Subsystem4 ==
  u : Inport
  Demux : Demux
  Mux : Mux
  Subsystem : Subsystem
  Subsystem1 : Subsystem
  Subsystem2 : Subsystem
  Subsystem3 : Subsystem
  Out1 : Outport
  wires:
  Subsystem2/1(Out1) -> Mux/3
  Demux/4 -> Subsystem3/1(u)
  Demux/3 -> Subsystem2/1(u)
  Subsystem1/1(Out1) -> Mux/2
  Demux/2 -> Subsystem1/1(u)
  Subsystem3/1(Out1) -> Mux/4
  Demux/1 -> Subsystem/1(u)
  Subsystem/1(Out1) -> Mux/1
  Mux/1 -> Out1/1
  u/1 -> Demux/1

== system simulation_Hippocampus_compare_paper/PDPD1/Controller/Subsystem1 ==
  x : Inport
  Demux1 : Demux  Outputs=12
  MATLAB Function : MATLAB Function  TreatAsAtomicUnit=on
  Mux1 : Mux  Inputs=12
  x_2pi : Outport
  wires:
  Mux1/1 -> x_2pi/1
  x/1 -> Demux1/1
  Demux1/6 -> MATLAB Function/1(u)
  Demux1/1 -> Mux1/1
  Demux1/2 -> Mux1/2
  Demux1/3 -> Mux1/3
  Demux1/4 -> Mux1/4
  Demux1/5 -> Mux1/5
  Demux1/7 -> Mux1/7
  Demux1/8 -> Mux1/8
  Demux1/9 -> Mux1/9
  Demux1/10 -> Mux1/10
  Demux1/11 -> Mux1/11
  Demux1/12 -> Mux1/12
  MATLAB Function/1(y) -> Mux1/6

== system simulation_Hippocampus_compare_paper/PDPD1/Disturbance: All derivatives1/disturbance2 ==
  Gain : Gain  Gain=[zeros(6,1);ones(6,1)]  Multiplication=Matrix(K*u)
  Step2 : Step  Time=60  After=0.5  SampleTime=0
  Step3 : Step  Time=55  After=0  SampleTime=0
  Sum1 : Sum
  Out1 : Outport
  wires:
  Step2/1 -> Sum1/1
  Step3/1 -> Sum1/2
  Gain/1 -> Out1/1
  Sum1/1 -> Gain/1

== system simulation_Hippocampus_compare_paper/PDPD1/Disturbance: All derivatives1/disturbance3 ==
  note: Subsystem
  a : Inport
  a1 : Inport  Port=2
  Constant : Constant  Value=10
  Constant2 : Constant  Value=10
  Constant3 : Constant  Value=45
  Constant4 : Constant  Value=20
  Gain : Gain  Gain=pi/180
  Gain1 : Gain  Gain=pi/180
  MATLAB Function : MATLAB Function  TreatAsAtomicUnit=on
  Mux : Mux  Inputs=3
  Subsystem1 : Subsystem
  d : Outport
  wires:
  Subsystem1/1(Out1) -> MATLAB Function/3(u_wave)
  Constant/1 -> MATLAB Function/5(u_un)
  Mux/1 -> MATLAB Function/4(u_c)
  MATLAB Function/1(d) -> d/1
  a1/1 -> MATLAB Function/1(p)
  a/1 -> MATLAB Function/2(a)
  Constant4/1 -> Mux/1
  Gain/1 -> Mux/2
  Gain1/1 -> Mux/3
  Constant3/1 -> Gain1/1
  Constant2/1 -> Gain/1

== system simulation_Hippocampus_compare_paper/PDPD1/Disturbance: All derivatives1/old disturbance ==
  Gain : Gain  Gain=ones(12,1)  Multiplication=Matrix(K*u)
  Step : Step  Time=50  After=0.5  SampleTime=0
  Step1 : Step  Time=55  After=-0.5  SampleTime=0
  Step2 : Step  Time=100  After=0.5  SampleTime=0
  Step3 : Step  Time=105  After=-0.5  SampleTime=0
  Sum : Sum  Inputs=|++
  Sum2 : Sum  Inputs=|++
  Sum3 : Sum  Inputs=|++
  Out1 : Outport
  wires:
  Gain/1 -> Out1/1
  Sum3/1 -> Gain/1
  Step3/1 -> Sum2/2
  Step/1 -> Sum/1
  Step1/1 -> Sum/2
  Step2/1 -> Sum2/1
  Sum/1 -> Sum3/1
  Sum2/1 -> Sum3/2

== system simulation_Hippocampus_compare_paper/PDPD1/HippCampus1/Subsystem ==
  In1 : Inport
  Demux : Demux  Outputs=[5 1 6]
  MATLAB Function : MATLAB Function  TreatAsAtomicUnit=on
  Mux : Mux  Inputs=3
  state : Outport
  wires:
  Demux/2 -> MATLAB Function/1(u)
  MATLAB Function/1(y) -> Mux/2
  In1/1 -> Demux/1
  Demux/3 -> Mux/3
  Demux/1 -> Mux/1
  Mux/1 -> state/1

== system simulation_Hippocampus_compare_paper/PDPD1/HippCampus1/Subsystem1 ==
  u : Inport
  Integrator2 : Integrator
  Sqrt1 : Sqrt
  norm1 : MATLAB Function  TreatAsAtomicUnit=on
  Out1 : Outport
  wires:
  norm1/1(y) -> Integrator2/1
  Sqrt1/1 -> Out1/1
  Integrator2/1 -> Sqrt1/1
  u/1 -> norm1/1(u)

== system simulation_Hippocampus_compare_paper/PDPD1/HippCampus1/Subsystem4 ==
  u : Inport
  Demux : Demux
  Mux : Mux
  Subsystem : Subsystem
  Subsystem1 : Subsystem
  Subsystem2 : Subsystem
  Subsystem3 : Subsystem
  Out1 : Outport
  wires:
  Subsystem2/1(Out1) -> Mux/3
  Demux/4 -> Subsystem3/1(u)
  Demux/3 -> Subsystem2/1(u)
  Subsystem1/1(Out1) -> Mux/2
  Demux/2 -> Subsystem1/1(u)
  Subsystem3/1(Out1) -> Mux/4
  Demux/1 -> Subsystem/1(u)
  Subsystem/1(Out1) -> Mux/1
  Mux/1 -> Out1/1
  u/1 -> Demux/1

== system simulation_Hippocampus_compare_paper/Proposed Linear gain/Controller/calculate derivative 1 ==
  In1 : Inport
  Clock : Clock
  Derivative : Derivative
  MATLAB Function : MATLAB Function  TreatAsAtomicUnit=on
  Saturation : Saturate  UpperLimit=[6;3;6;6]  LowerLimit=-[6;3;6;6]
  y : Outport
  wires:
  Clock/1 -> MATLAB Function/2(t)
  In1/1 -> Derivative/1
  MATLAB Function/1(y) -> Saturation/1
  Derivative/1 -> MATLAB Function/1(u)
  Saturation/1 -> y/1

== system simulation_Hippocampus_compare_paper/Proposed Linear gain/Disturbance: All derivatives1/disturbance2 ==
  Gain : Gain  Gain=[0;0;0;0;0;0;1;1;1;1;1;1]  Multiplication=Matrix(K*u)
  Step2 : Step  Time=60  After=0.5  SampleTime=0
  Step3 : Step  Time=55  After=0  SampleTime=0
  Sum1 : Sum  Inputs=-+
  Out1 : Outport
  wires:
  Step2/1 -> Sum1/1
  Step3/1 -> Sum1/2
  Gain/1 -> Out1/1
  Sum1/1 -> Gain/1

== system simulation_Hippocampus_compare_paper/Proposed Linear gain/Disturbance: All derivatives1/disturbance3 ==
  note: Subsystem
  a : Inport
  a1 : Inport  Port=2
  Constant : Constant  Value=10
  Constant2 : Constant  Value=10
  Constant3 : Constant  Value=45
  Constant4 : Constant  Value=20
  Gain : Gain  Gain=pi/180
  Gain1 : Gain  Gain=pi/180
  MATLAB Function : MATLAB Function  TreatAsAtomicUnit=on
  Mux : Mux  Inputs=3
  Subsystem1 : Subsystem
  d : Outport
  wires:
  Subsystem1/1(Out1) -> MATLAB Function/3(u_wave)
  Constant/1 -> MATLAB Function/5(u_un)
  Mux/1 -> MATLAB Function/4(u_c)
  MATLAB Function/1(d) -> d/1
  a1/1 -> MATLAB Function/1(p)
  a/1 -> MATLAB Function/2(a)
  Constant4/1 -> Mux/1
  Gain/1 -> Mux/2
  Gain1/1 -> Mux/3
  Constant3/1 -> Gain1/1
  Constant2/1 -> Gain/1

== system simulation_Hippocampus_compare_paper/Proposed Linear gain/Disturbance: All derivatives1/old disturbance ==
  Gain : Gain  Gain=ones(12,1)  Multiplication=Matrix(K*u)
  Step : Step  Time=50  After=0.5  SampleTime=0
  Step1 : Step  Time=55  After=-0.5  SampleTime=0
  Step2 : Step  Time=100  After=0.5  SampleTime=0
  Step3 : Step  Time=105  After=-0.5  SampleTime=0
  Sum : Sum  Inputs=|++
  Sum2 : Sum  Inputs=|++
  Sum3 : Sum  Inputs=|++
  Out1 : Outport
  wires:
  Gain/1 -> Out1/1
  Sum3/1 -> Gain/1
  Step3/1 -> Sum2/2
  Step/1 -> Sum/1
  Step1/1 -> Sum/2
  Step2/1 -> Sum2/1
  Sum/1 -> Sum3/1
  Sum2/1 -> Sum3/2

== system simulation_Hippocampus_compare_paper/Proposed Linear gain/Disturbance: All derivatives2/disturbance2 ==
  Gain : Gain  Gain=[0;0;0;0;0;0;1;1;1;1;1;1]  Multiplication=Matrix(K*u)
  Step2 : Step  Time=60  After=0.5  SampleTime=0
  Step3 : Step  Time=55  After=0  SampleTime=0
  Sum1 : Sum
  Out1 : Outport
  wires:
  Step2/1 -> Sum1/1
  Step3/1 -> Sum1/2
  Gain/1 -> Out1/1
  Sum1/1 -> Gain/1
